simulink model "doublePendumSimulation"  (R2022b)
settings: Solver=VariableStepAuto  StartTime=0.0  StopTime=T  MaxStep=0.00001  RelTol=1e-3
values from neighbouring files (symbols this model uses):
  g = 9.81    [variables.m]
  l1 = 0.3    [variables.m]
  l2 = 0.25    [variables.m]
  m1 = 0.2    [variables.m]
  m2 = 0.1    [variables.m]
settings Model: Creator=Cris  LastModifiedBy=Cris

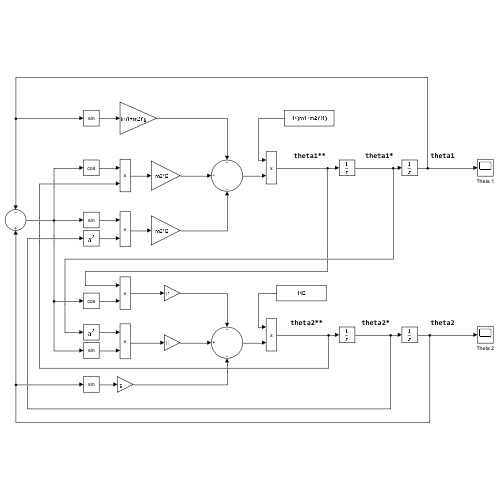
[thumbnail: Simulink's stored preview of the top-level diagram]
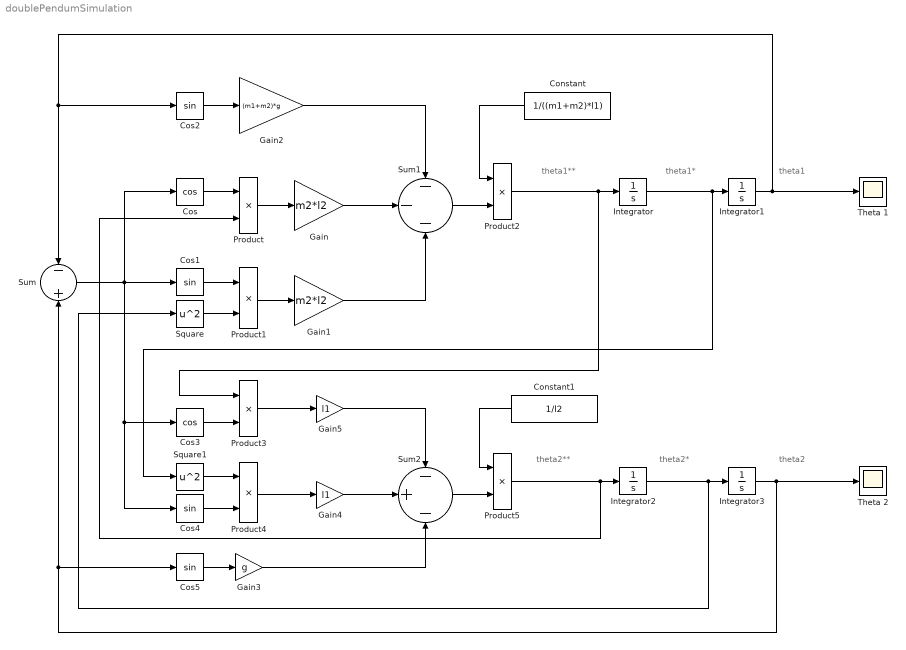
== system doublePendumSimulation ==
  note: theta1**
  note: theta1*
  note: theta1
  note: theta2**
  note: theta2*
  note: theta2
  Constant : Constant  Value=1/((m1+m2)*l1)
  Constant1 : Constant  Value=1/l2
  Cos : Trigonometry  Operator=cos
  Cos{1..2,4..5} (4 alike) : Trigonometry
  Cos3 : Trigonometry  Operator=cos
  Gain : Gain  Gain=m2*l2
  Gain1 : Gain  Gain=m2*l2
  Gain2 : Gain  Gain=(m1+m2)*g
  Gain3 : Gain  Gain=g
  Gain4 : Gain  Gain=l1
  Gain5 : Gain  Gain=l1
  Integrator : Integrator
  Integrator1 : Integrator
  Integrator2 : Integrator
  Integrator3 : Integrator  InitialCondition=35*pi/180
  Product{,1..5} (6 alike) : Product
  Square : Math  Operator=square
  Square1 : Math  Operator=square
  Sum : Sum  Inputs=-+
  Sum1 : Sum  Inputs=---
  Sum2 : Sum  Inputs=-+-
  Theta 1 : Scope
  Theta 2 : Scope
  wires:
  Sum/1 -> Cos3/1, Cos4/1, Cos1/1, Cos/1
  Cos/1 -> Product/1
  Cos1/1 -> Product1/1
  Square/1 -> Product1/2
  Product/1 -> Gain/1
  Product1/1 -> Gain1/1
  Cos2/1 -> Gain2/1
  Gain1/1 -> Sum1/3
  Gain/1 -> Sum1/2
  Gain2/1 -> Sum1/1
  Integrator/1 -> Square1/1, Integrator1/1
  Integrator1/1 -> Theta 1/1, Sum/1, Cos2/1
  Sum1/1 -> Product2/2
  Product2/1 -> Product3/1, Integrator/1
  Constant/1 -> Product2/1
  Cos3/1 -> Product3/2
  Cos5/1 -> Gain3/1
  Product4/1 -> Gain4/1
  Product3/1 -> Gain5/1
  Gain3/1 -> Sum2/3
  Square1/1 -> Product4/1
  Cos4/1 -> Product4/2
  Gain4/1 -> Sum2/2
  Gain5/1 -> Sum2/1
  Sum2/1 -> Product5/2
  Constant1/1 -> Product5/1
  Product5/1 -> Product/2, Integrator2/1
  Integrator2/1 -> Square/1, Integrator3/1
  Integrator3/1 -> Theta 2/1, Cos5/1, Sum/2
